simulink model "SETL3_TestLevel_3_MODEL_Training"  (R2017b)
settings: Solver=VariableStepAuto  StartTime=0.0  StopTime=20000000  RelTol=1e-3
libraries: instrumentlib x2, svdutilitieslib x1
settings Model: Creator=Bruger  LastModifiedBy=koch

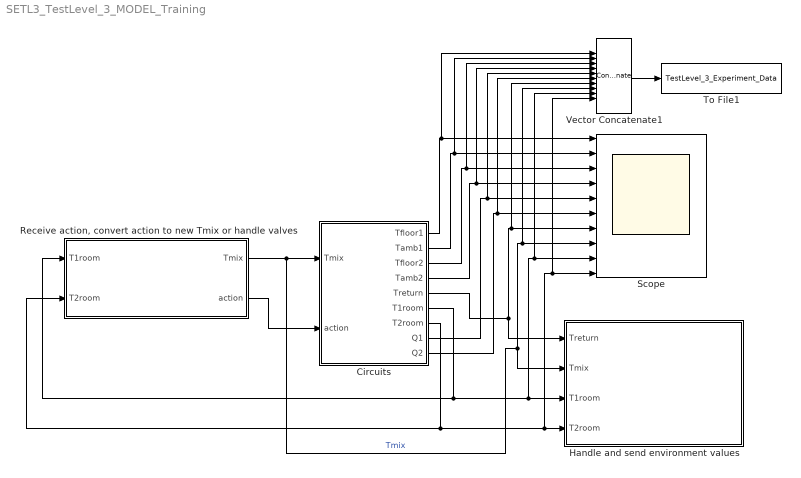
== system SETL3_TestLevel_3_MODEL_Training ==
  Circuits : Subsystem
  Handle and send environment values : Subsystem
  "Receive action, convert action to new Tmix or handle valves" : Subsystem
  Scope : Scope  NumInputPorts=10
  To File1 : ToFile  Filename=TestLevel_3_Experiment_Data  SaveFormat=Timeseries
  Vector Concatenate1 : Concatenate  NumInputs=10
  wires:
  Vector Concatenate1/1 -> To File1/1
  "Receive action, convert action to new Tmix or handle valves"/1(Tmix) -> Vector Concatenate1/8, Scope/8, Handle and send environment values/2(Tmix), Circuits/1(Tmix)  "Tmix"
  Circuits/7(T2room) -> Vector Concatenate1/10, Scope/10, Handle and send environment values/4(T2room), "Receive action, convert action to new Tmix or handle valves"/2(T2room)
  Circuits/6(T1room) -> Vector Concatenate1/9, Scope/9, Handle and send environment values/3(T1room), "Receive action, convert action to new Tmix or handle valves"/1(T1room)
  Circuits/1(Tfloor1) -> Vector Concatenate1/1, Scope/1
  Circuits/2(Tamb1) -> Vector Concatenate1/2, Scope/2
  Circuits/3(Tfloor2) -> Vector Concatenate1/3, Scope/3
  Circuits/4(Tamb2) -> Vector Concatenate1/4, Scope/4
  Circuits/8(Q1) -> Vector Concatenate1/5, Scope/5
  Circuits/9(Q2) -> Vector Concatenate1/6, Scope/6
  "Receive action, convert action to new Tmix or handle valves"/2(action) -> Circuits/2(action)
  Circuits/5(Treturn) -> Vector Concatenate1/7, Scope/7, Handle and send environment values/1(Treturn)

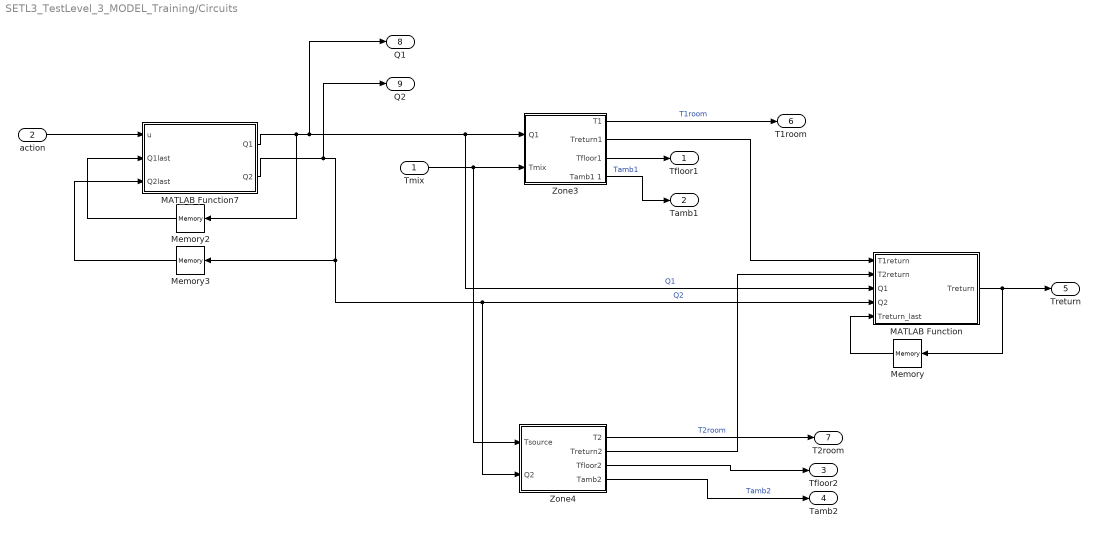
== system SETL3_TestLevel_3_MODEL_Training/Circuits ==
  Tmix : Inport
  action : Inport  Port=2
  MATLAB Function : MATLAB Function  TreatAsAtomicUnit=on
  MATLAB Function7 : MATLAB Function  TreatAsAtomicUnit=on
  Memory : Memory
  Memory2 : Memory  InitialCondition=0.000027777778
  Memory3 : Memory  InitialCondition=0.000027777778
  Zone3 : Subsystem  Tag=Zone1  Description=Zone1
  Zone4 : Subsystem
  Tfloor1 : Outport
  Tamb1 : Outport  Port=2
  Tfloor2 : Outport  Port=3
  Tamb2 : Outport  Port=4
  Treturn : Outport  Port=5
  T1room : Outport  Port=6
  T2room : Outport  Port=7
  Q1 : Outport  Port=8
  Q2 : Outport  Port=9
  wires:
  MATLAB Function/1(Treturn) -> Memory/1, Treturn/1
  Zone4/3("Tfloor2 ") -> Tfloor2/1
  Zone3/3("Tfloor1 ") -> Tfloor1/1
  Zone4/4(Tamb2) -> Tamb2/1  "Tamb2"
  Zone3/4(Tamb1 1) -> Tamb1/1  "Tamb1"
  Tmix/1 -> Zone4/1(Tsource), Zone3/2(Tmix)
  action/1 -> MATLAB Function7/1(u)
  Zone4/2("Treturn2 ") -> MATLAB Function/2(T2return)
  Zone3/2("Treturn1 ") -> MATLAB Function/1(T1return)
  Zone3/1(T1) -> T1room/1  "T1room"
  Zone4/1("T2 ") -> T2room/1  "T2room"
  MATLAB Function7/1(Q1) -> Memory2/1, Zone3/1("Q1 "), MATLAB Function/3(Q1), Q1/1  "Q1"
  MATLAB Function7/2(Q2) -> Zone4/2("Q2 "), MATLAB Function/4(Q2), Memory3/1, Q2/1  "Q2"
  Memory2/1 -> MATLAB Function7/2(Q1last)
  Memory3/1 -> MATLAB Function7/3(Q2last)
  Memory/1 -> MATLAB Function/5(Treturn_last)

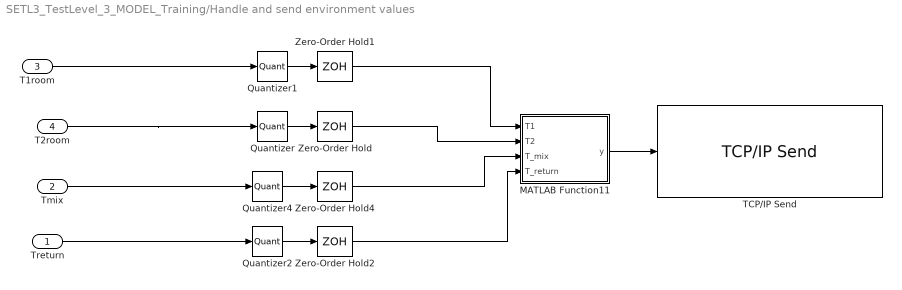
== system SETL3_TestLevel_3_MODEL_Training/Handle and send environment values ==
  Treturn : Inport
  Tmix : Inport  Port=2
  T1room : Inport  Port=3
  T2room : Inport  Port=4
  MATLAB Function11 : MATLAB Function  TreatAsAtomicUnit=on
  Quantizer{,1..2,4} (4 alike) : Quantizer  QuantizationInterval=0.01
  TCP/IP Send : instrumentlib/TCP//IP Send  Priority=2  Host=localhost  Port=50001  EnableBlockingMode=on  Timeout=40  ByteOrder=LittleEndian
      settings: SourceProductName=Instrument Control Toolbox
  Zero-Order Hold{,1..2,4} (4 alike) : ZeroOrderHold  SampleTime=-1
  wires:
  T2room/1 -> Quantizer/1
  Tmix/1 -> Quantizer4/1
  T1room/1 -> Quantizer1/1
  Zero-Order Hold2/1 -> MATLAB Function11/4(T_return)
  Quantizer2/1 -> Zero-Order Hold2/1
  Zero-Order Hold1/1 -> MATLAB Function11/1(T1)
  Quantizer1/1 -> Zero-Order Hold1/1
  MATLAB Function11/1(y) -> TCP/IP Send/1
  Zero-Order Hold/1 -> MATLAB Function11/2(T2)
  Quantizer/1 -> Zero-Order Hold/1
  Quantizer4/1 -> Zero-Order Hold4/1
  Zero-Order Hold4/1 -> MATLAB Function11/3(T_mix)
  Treturn/1 -> Quantizer2/1

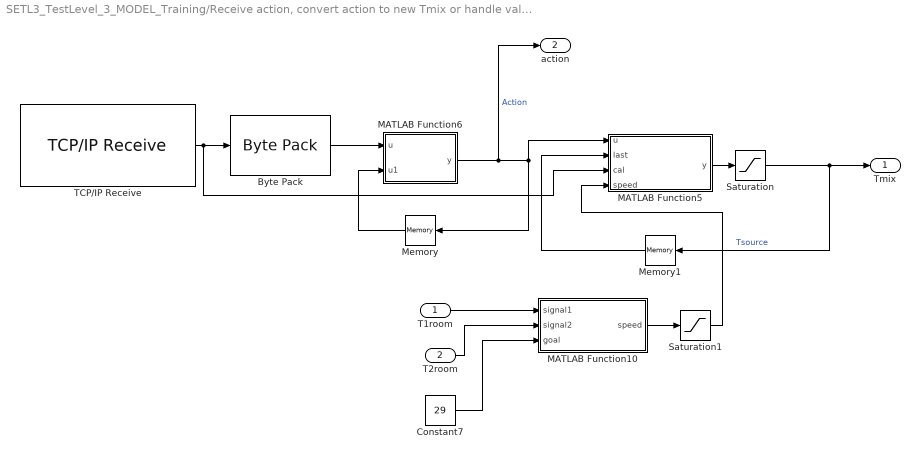
== system SETL3_TestLevel_3_MODEL_Training/Receive action, convert action to new Tmix or handle valves ==
  T1room : Inport
  T2room : Inport  Port=2
  Byte Pack : svdutilitieslib/Byte Pack  datatypes={'uint8'}  byteAlign=1  blockPlatform=arduinoert
      settings: SourceProductName=Simulink Support Package for Arduino Hardware  SourceProductBaseCode=ARDUINO
  Constant7 : Constant  Value=29
  MATLAB Function10 : MATLAB Function  TreatAsAtomicUnit=on
  MATLAB Function5 : MATLAB Function  TreatAsAtomicUnit=on
  MATLAB Function6 : MATLAB Function  TreatAsAtomicUnit=on
  Memory : Memory
  Memory1 : Memory  InitialCondition=24
  Saturation : Saturate  UpperLimit=60  LowerLimit=24
  Saturation1 : Saturate  UpperLimit=0.8  LowerLimit=0.005
  TCP/IP Receive : instrumentlib/TCP//IP Receive  Host=localhost  Port=50000  DataSize=[1 1]  EnableBlockingMode=on  Timeout=80  SampleTime=50  DataType=uint8  ByteOrder=BigEndian
      settings: SourceProductName=Instrument Control Toolbox
  Tmix : Outport
  action : Outport  Port=2
  wires:
  T1room/1 -> MATLAB Function10/1(signal1)
  T2room/1 -> MATLAB Function10/2(signal2)
  MATLAB Function5/1(y) -> Saturation/1
  Memory/1 -> MATLAB Function6/2(u1)
  Constant7/1 -> MATLAB Function10/3(goal)
  Saturation1/1 -> MATLAB Function5/4(speed)
  Byte Pack/1 -> MATLAB Function6/1(u)
  MATLAB Function10/1(speed) -> Saturation1/1
  Memory1/1 -> MATLAB Function5/2(last)
  TCP/IP Receive/1 -> MATLAB Function5/3(cal), Byte Pack/1
  MATLAB Function6/1(y) -> action/1, MATLAB Function5/1(u), Memory/1  "Action"
  Saturation/1 -> Memory1/1, Tmix/1  "Tsource"

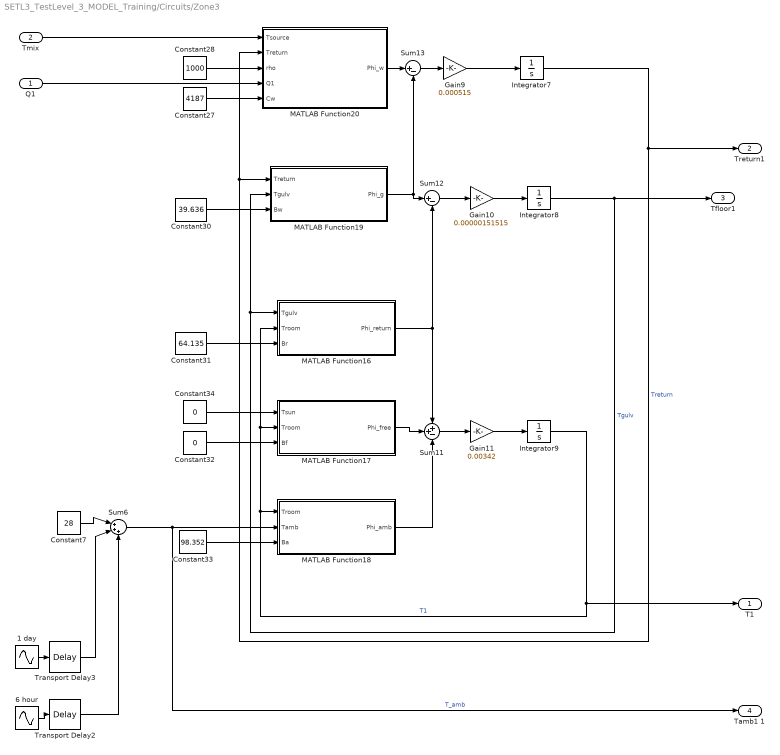
== system SETL3_TestLevel_3_MODEL_Training/Circuits/Zone3 ==
  "Q1 " : Inport
  Tmix : Inport  Port=2
  1 day : Sin  Frequency=0.00007272205216643  SampleTime=0
  6 hour : Sin  Frequency=0.010471975  SampleTime=0
  Constant27 : Constant  Value=4187
  Constant28 : Constant  Value=1000
  Constant30 : Constant  Value=39.636
  Constant31 : Constant  Value=64.135
  Constant32 : Constant  Value=0
  Constant33 : Constant  Value=98.352
  Constant34 : Constant  Value=0
  Constant7 : Constant  Value=28
  Gain10 : Gain  Gain=0.00000151515
  Gain11 : Gain  Gain=0.00342
  Gain9 : Gain  Gain=0.000515
  Integrator7 : Integrator  InitialCondition=15
  Integrator8 : Integrator  InitialCondition=15
  Integrator9 : Integrator  InitialCondition=15
  MATLAB Function16 : MATLAB Function  TreatAsAtomicUnit=on
  MATLAB Function17 : MATLAB Function  TreatAsAtomicUnit=on
  MATLAB Function18 : MATLAB Function  TreatAsAtomicUnit=on
  MATLAB Function19 : MATLAB Function  TreatAsAtomicUnit=on
  MATLAB Function20 : MATLAB Function  TreatAsAtomicUnit=on
  Sum11 : Sum  Inputs=++-
  Sum12 : Sum  Inputs=|+-
  Sum13 : Sum  Inputs=|+-
  Sum6 : Sum  Inputs=|+++
  Transport Delay2 : TransportDelay  DelayTime=4000000
  Transport Delay3 : TransportDelay  DelayTime=3000000
  T1 : Outport
  "Treturn1 " : Outport  Port=2
  "Tfloor1 " : Outport  Port=3
  Tamb1 1 : Outport  Port=4
  wires:
  Tmix/1 -> MATLAB Function20/1(Tsource)
  MATLAB Function20/1(Phi_w) -> Sum13/1
  Sum12/1 -> Gain10/1
  Constant31/1 -> MATLAB Function16/3(Br)
  Constant32/1 -> MATLAB Function17/3(Bf)
  Integrator7/1 -> "Treturn1 "/1, MATLAB Function20/2(Treturn), MATLAB Function19/1(Treturn)  "Treturn"
  Gain11/1 -> Integrator9/1
  Constant33/1 -> MATLAB Function18/3(Ba)
  Gain9/1 -> Integrator7/1
  Constant34/1 -> MATLAB Function17/1(Tsun)
  Constant30/1 -> MATLAB Function19/3(Bw)
  Constant27/1 -> MATLAB Function20/5(Cw)
  Integrator9/1 -> MATLAB Function16/2(Troom), MATLAB Function17/2(Troom), MATLAB Function18/1(Troom), T1/1  "T1"
  MATLAB Function18/1(Phi_amb) -> Sum11/3
  MATLAB Function19/1(Phi_g) -> Sum13/2, Sum12/1
  Sum11/1 -> Gain11/1
  Sum13/1 -> Gain9/1
  Integrator8/1 -> "Tfloor1 "/1, MATLAB Function16/1(Tgulv), MATLAB Function19/2(Tgulv)  "Tgulv"
  MATLAB Function16/1(Phi_return) -> Sum11/1, Sum12/2
  MATLAB Function17/1(Phi_free) -> Sum11/2
  Gain10/1 -> Integrator8/1
  Constant28/1 -> MATLAB Function20/3(rho)
  "Q1 "/1 -> MATLAB Function20/4(Q1)
  Sum6/1 -> Tamb1 1/1, MATLAB Function18/2(Tamb)  "T_amb"
  Constant7/1 -> Sum6/1
  Transport Delay2/1 -> Sum6/3
  Transport Delay3/1 -> Sum6/2
  6 hour/1 -> Transport Delay2/1
  1 day/1 -> Transport Delay3/1

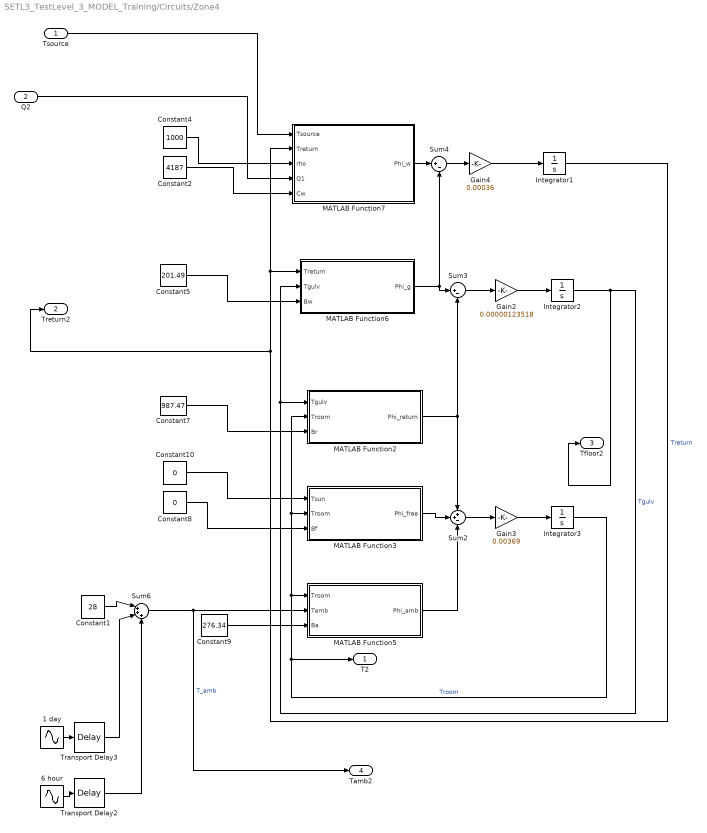
== system SETL3_TestLevel_3_MODEL_Training/Circuits/Zone4 ==
  Tsource : Inport
  "Q2 " : Inport  Port=2
  1 day : Sin  Frequency=0.00007272205216643  SampleTime=0
  6 hour : Sin  Frequency=0.010471975  SampleTime=0
  Constant1 : Constant  Value=28
  Constant10 : Constant  Value=0
  Constant2 : Constant  Value=4187
  Constant4 : Constant  Value=1000
  Constant5 : Constant  Value=201.49
  Constant7 : Constant  Value=987.47
  Constant8 : Constant  Value=0
  Constant9 : Constant  Value=276.34
  Gain2 : Gain  Gain=0.00000123518
  Gain3 : Gain  Gain=0.00369
  Gain4 : Gain  Gain=0.00036
  Integrator1 : Integrator  InitialCondition=15
  Integrator2 : Integrator  InitialCondition=15
  Integrator3 : Integrator  InitialCondition=15
  MATLAB Function2 : MATLAB Function  TreatAsAtomicUnit=on
  MATLAB Function3 : MATLAB Function  TreatAsAtomicUnit=on
  MATLAB Function5 : MATLAB Function  TreatAsAtomicUnit=on
  MATLAB Function6 : MATLAB Function  TreatAsAtomicUnit=on
  MATLAB Function7 : MATLAB Function  TreatAsAtomicUnit=on
  Sum2 : Sum  Inputs=++-
  Sum3 : Sum  Inputs=|+-
  Sum4 : Sum  Inputs=|+-
  Sum6 : Sum  Inputs=|+++
  Transport Delay2 : TransportDelay  DelayTime=4000000
  Transport Delay3 : TransportDelay  DelayTime=3000000
  "T2 " : Outport
  "Treturn2 " : Outport  Port=2
  "Tfloor2 " : Outport  Port=3
  Tamb2 : Outport  Port=4
  wires:
  Gain4/1 -> Integrator1/1
  Gain3/1 -> Integrator3/1
  MATLAB Function5/1(Phi_amb) -> Sum2/3
  Integrator2/1 -> "Tfloor2 "/1, MATLAB Function2/1(Tgulv), MATLAB Function6/2(Tgulv)  "Tgulv"
  Constant2/1 -> MATLAB Function7/5(Cw)
  MATLAB Function7/1(Phi_w) -> Sum4/1
  Sum4/1 -> Gain4/1
  Sum3/1 -> Gain2/1
  Integrator1/1 -> MATLAB Function7/2(Treturn), MATLAB Function6/1(Treturn), "Treturn2 "/1  "Treturn"
  Gain2/1 -> Integrator2/1
  MATLAB Function2/1(Phi_return) -> Sum2/1, Sum3/2
  Constant7/1 -> MATLAB Function2/3(Br)
  MATLAB Function6/1(Phi_g) -> Sum4/2, Sum3/1
  MATLAB Function3/1(Phi_free) -> Sum2/2
  Constant9/1 -> MATLAB Function5/3(Ba)
  Constant4/1 -> MATLAB Function7/3(rho)
  Integrator3/1 -> MATLAB Function2/2(Troom), MATLAB Function3/2(Troom), MATLAB Function5/1(Troom), "T2 "/1  "Troom"
  Sum2/1 -> Gain3/1
  Constant5/1 -> MATLAB Function6/3(Bw)
  "Q2 "/1 -> MATLAB Function7/4(Q1)
  Constant8/1 -> MATLAB Function3/3(Bf)
  Constant10/1 -> MATLAB Function3/1(Tsun)
  Tsource/1 -> MATLAB Function7/1(Tsource)
  Sum6/1 -> Tamb2/1, MATLAB Function5/2(Tamb)  "T_amb"
  Constant1/1 -> Sum6/1
  Transport Delay2/1 -> Sum6/3
  Transport Delay3/1 -> Sum6/2
  6 hour/1 -> Transport Delay2/1
  1 day/1 -> Transport Delay3/1

== matlab function SETL3_TestLevel_3_MODEL_Training/Receive action, convert action to new Tmix or handle valves/MATLAB Function5 ==
  data: u input; y output; last input; cal input; speed input
function y = fcn(u,last,cal,speed)

    if cal > 0 
         k=1

    else
         k=0
    end


if u < 2 && k>0
y = last
k=0
elseif 1 < u && u < 3 && k>0
    y=last - speed
    k=0
elseif 2 < u && k>0 && u < 4
    y = last+speed
    k=0
elseif u > 20
    y = u;
else
    y=last
   
end

== matlab function SETL3_TestLevel_3_MODEL_Training/Receive action, convert action to new Tmix or handle valves/MATLAB Function6 ==
  data: u input; y output; u1 input
function y  = fcn(u,u1)

u = double(u);
% zero is not a option so
if u > 0
    y = u;
else
    y = u1;
end

== matlab function SETL3_TestLevel_3_MODEL_Training/Circuits/Zone4/MATLAB Function2 ==
  data: Tgulv input; Phi_return output; Troom input; Br input
function Phi_return = fcn(Tgulv,Troom,Br)

Phi_return = Br * ( Tgulv-Troom)

== matlab function SETL3_TestLevel_3_MODEL_Training/Circuits/Zone4/MATLAB Function3 ==
  data: Tsun input; Phi_free output; Troom input; Bf input
function Phi_free = fcn(Tsun,Troom,Bf)

Phi_free = Bf * ( Tsun-Troom)

== matlab function SETL3_TestLevel_3_MODEL_Training/Circuits/MATLAB Function7 ==
  data: u input; Q1 output; Q2 output; Q1last input; Q2last input
function [Q1,Q2]= fcn(u,Q1last,Q2last)
    
if u < 4 || (u > 20)
    Q1 = Q1last
    Q2 = Q2last
elseif u > 3 && 5 > u
    Q1 = 0.0001875
    Q2 = 0.0001875
elseif u > 4 && 6 > u
    Q1 = 0.00025
    Q2 = 0
elseif u > 5 && 7 > u
    Q1 = 0
    Q2 = 0.00025
elseif u > 6 && 8 > u
    Q1 = 0
    Q2 = 0
else 
    Q1 = 0
    Q2 = 0
end

== matlab function SETL3_TestLevel_3_MODEL_Training/Circuits/Zone4/MATLAB Function5 ==
  data: Troom input; Tamb input; Phi_amb output; Ba input
function Phi_amb = fcn(Troom,Tamb,Ba)

Phi_amb = Ba * ( Troom-Tamb)

== matlab function SETL3_TestLevel_3_MODEL_Training/Circuits/Zone4/MATLAB Function6 ==
  data: Treturn input; Tgulv input; Phi_g output; Bw input
function Phi_g= fcn(Treturn,Tgulv,Bw)

Phi_g = Bw * ( Treturn-Tgulv)

== matlab function SETL3_TestLevel_3_MODEL_Training/Circuits/Zone4/MATLAB Function7 ==
  data: Tsource input; Treturn input; Phi_w output; rho input; Q1 input; Cw input
function Phi_w= fcn(Tsource,Treturn,rho,Q1,Cw)

Phi_w = rho*Q1*0.8 *Cw* ( Tsource-Treturn)

== matlab function SETL3_TestLevel_3_MODEL_Training/Circuits/MATLAB Function ==
  data: T1return input; Treturn output; T2return input; Q1 input; Q2 input; Treturn_last input
function Treturn = fcn(T1return, T2return, Q1, Q2, Treturn_last)

Treturn = (T1return * (Q1/(Q1+Q2))) + (T2return * (Q2/(Q1+Q2)));

if Q1 < 0.0000001 && Q2 < 0.0000001
    Treturn = Treturn_last;
end

== matlab function SETL3_TestLevel_3_MODEL_Training/Receive action, convert action to new Tmix or handle valves/MATLAB Function10 ==
  data: speed output; signal1 input; signal2 input; goal input
function speed = fcn(signal1,signal2, goal)

delta1 =abs(goal - signal1)
delta2 =abs(goal - signal2)

Delta = [delta1;delta2]

if goal > 0 && signal1 > 0
speed = min(Delta)*0.3
else 
    speed = 0.1
end

if speed < 0.03
    speed =0.03
end

== matlab function SETL3_TestLevel_3_MODEL_Training/Handle and send environment values/MATLAB Function11 ==
  data: T1 input; T2 input; y output; T_mix input; T_return input
function y = fcn(T1, T2, T_mix, T_return)


y = [T1, T2, 4.6, 4.7, T_mix, T_return];

== matlab function SETL3_TestLevel_3_MODEL_Training/Circuits/Zone3/MATLAB Function16 ==
  data: Tgulv input; Phi_return output; Troom input; Br input
function Phi_return = fcn(Tgulv,Troom,Br)

Phi_return = Br * ( Tgulv-Troom)

== matlab function SETL3_TestLevel_3_MODEL_Training/Circuits/Zone3/MATLAB Function17 ==
  data: Tsun input; Phi_free output; Troom input; Bf input
function Phi_free = fcn(Tsun,Troom,Bf)

Phi_free = Bf * ( Tsun-Troom)

== matlab function SETL3_TestLevel_3_MODEL_Training/Circuits/Zone3/MATLAB Function18 ==
  data: Troom input; Tamb input; Phi_amb output; Ba input
function Phi_amb = fcn(Troom,Tamb,Ba)

Phi_amb = Ba * ( Troom-Tamb)

== matlab function SETL3_TestLevel_3_MODEL_Training/Circuits/Zone3/MATLAB Function19 ==
  data: Treturn input; Tgulv input; Phi_g output; Bw input
function Phi_g= fcn(Treturn,Tgulv,Bw)

Phi_g = Bw * ( Treturn-Tgulv)

== matlab function SETL3_TestLevel_3_MODEL_Training/Circuits/Zone3/MATLAB Function20 ==
  data: Tsource input; Treturn input; Phi_w output; rho input; Q1 input; Cw input
function Phi_w= fcn(Tsource,Treturn,rho,Q1,Cw)

Phi_w = rho*Q1 *Cw* ( Tsource-Treturn)
